simulink model "SOFIE_github_18"  (R2018a)
settings: Solver=FixedStepAuto  StartTime=0.0  StopTime=12  FixedStep=5e-6  MinStep=1e-5  RelTol=1e-3
undefined symbols (not defined in the file): start
libraries: powerlib x13, powerlib_meascontrol x5
settings Model: Creator=110198  LastModifiedBy=malinche
settings DataIOCC: ReturnWorkspaceOutputs=on
settings SFSimCC: SimUseLocalCustomCode=on
settings RTWCC: RTWUseLocalCustomCode=on

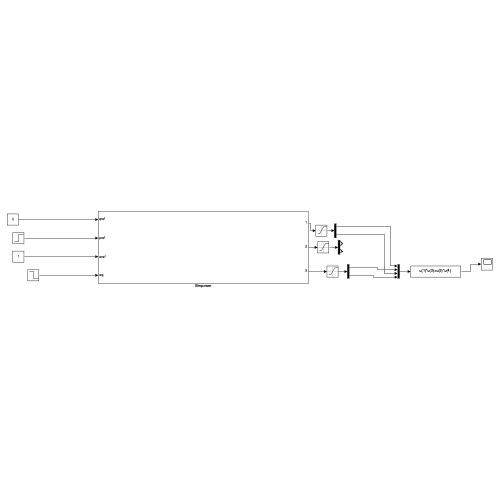
[thumbnail: Simulink's stored preview of the top-level diagram]
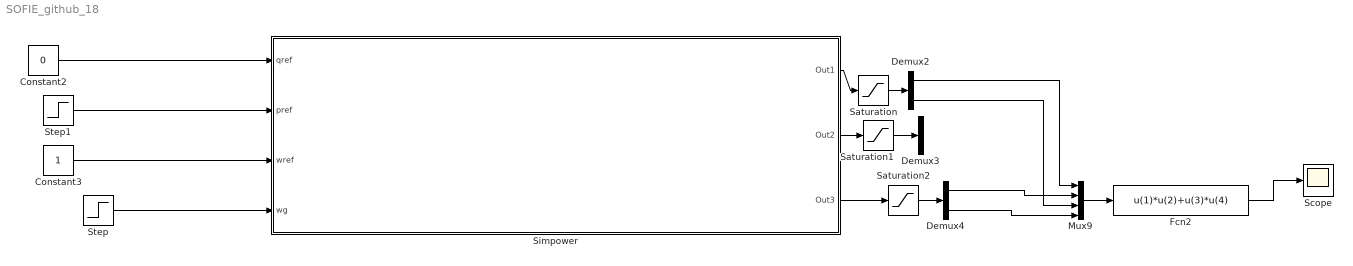
== system SOFIE_github_18 ==
  Constant2 : Constant  Value=0
  Constant3 : Constant
  Demux2 : Demux  Outputs=2
  Demux3 : Demux  Outputs=2
  Demux4 : Demux  Outputs=2
  Fcn2 : Fcn  Expr=u(1)*u(2)+u(3)*u(4)
  Mux9 : Mux
  Saturation : Saturate  UpperLimit=1.5  LowerLimit=-1.5
  Saturation1 : Saturate  UpperLimit=1.5  LowerLimit=-1.5
  Saturation2 : Saturate  UpperLimit=1.5  LowerLimit=-1.5
  Scope : Scope
  Simpower : Subsystem
  Step : Step  Time=4  Before=1  After=1-0.01  SampleTime=0
  Step1 : Step  Time=8  After=0.1  SampleTime=0
  wires:
  Step1/1 -> Simpower/2(pref)
  Constant2/1 -> Simpower/1(qref)
  Step/1 -> Simpower/4(wg)
  Constant3/1 -> Simpower/3(wref)
  Simpower/1(Out1) -> Saturation/1
  Demux2/1 -> Mux9/1
  Demux2/2 -> Mux9/3
  Simpower/2(Out2) -> Saturation1/1
  Saturation/1 -> Demux2/1
  Saturation1/1 -> Demux3/1
  Saturation2/1 -> Demux4/1
  Simpower/3(Out3) -> Saturation2/1
  Demux4/1 -> Mux9/2
  Demux4/2 -> Mux9/4
  Mux9/1 -> Fcn2/1
  Fcn2/1 -> Scope/1

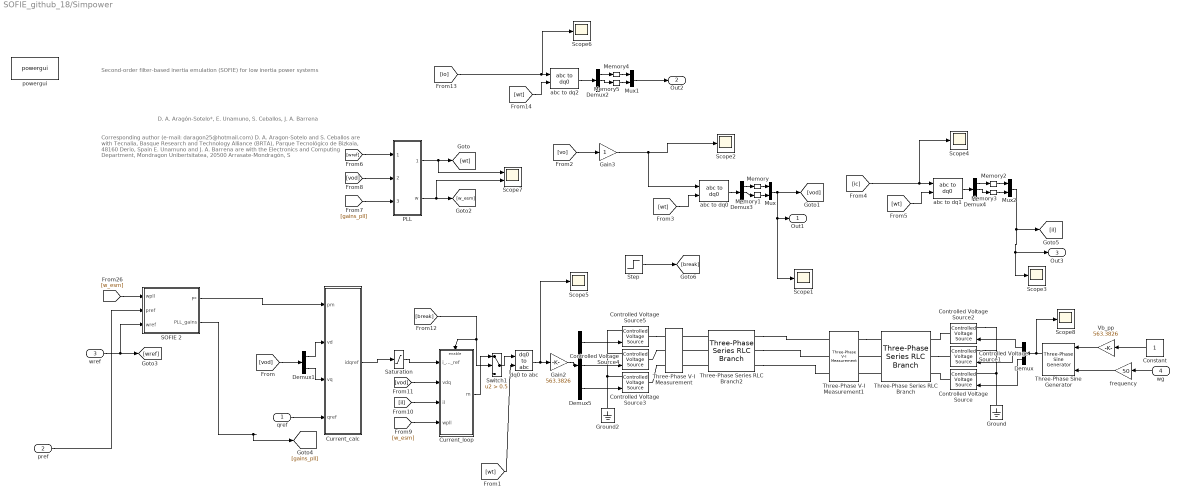
== system SOFIE_github_18/Simpower ==
  note: Second-order filter-based inertia emulation
      | (SOFIE) for low inertia power systems
  note: Corresponding author (e-mail: daragon25@hotmail.com)
      | D. A. Aragon-Sotelo and S. Ceballos are with Tecnalia, Basque Research
      | and Technology Alliance (BRTA), Parque Tecnológico de Bizkaia, 48160
      | Derio, Spain
      | E. Unamuno and J. A. Barrena are with the Electronics and Computing
      | Department, Mondragon Unibertsitatea, 20500 Arrasate-Mondragón, S
  note: D. A. Aragón-Sotelo*, E. Unamuno, S. Ceballos, J. A. Barrena
  qref : Inport
  pref : Inport  Port=2
  wref : Inport  Port=3
  wg : Inport  Port=4
  Constant : Constant
  Controlled Voltage Source{,1..5} (6 alike) : powerlib/Electrical Sources/Controlled Voltage Source  Initialize=off  Source_Type=AC  Amplitude=0  Phase=0  Frequency=0  Measurements=None
  Current_calc : Subsystem
  Current_loop : Subsystem
  Demux{,2..5} (5 alike) : Demux  Outputs=3
  Demux1 : Demux  Outputs=2
  Gain2 : Gain  Gain=563.3826
  Gain3 : Gain
  Ground : powerlib/Elements/Ground  LConnTagsString=a
  Ground2 : powerlib/Elements/Ground  LConnTagsString=a
  Memory : Memory  InitialCondition=1
  Memory1 : Memory
  Memory2 : Memory  InitialCondition=1
  Memory3 : Memory
  Memory4 : Memory  InitialCondition=1
  Memory5 : Memory
  Mux : Mux  Inputs=2
  Mux1 : Mux  Inputs=2
  Mux2 : Mux  Inputs=2
  PLL : Subsystem
  SOFIE 2 : Subsystem
  Saturation : Saturate  UpperLimit=2  LowerLimit=-2
  Scope{1..6,8} (7 alike) : Scope
  Scope7 : Scope  NumInputPorts=2
  Step : Step  Time=2  SampleTime=0
  Switch1 : Switch  Criteria=u2 > Threshold  Threshold=0.5
  Three-Phase Series RLC Branch : powerlib/Elements/Three-Phase Series RLC Branch  LConnTagsString=A|B|C  RConnTagsString=A|B|C  BranchType=RL  Resistance=0.0017  Inductance=1.6532e-05  Capacitance=1e-6  Measurements=None
  Three-Phase Series RLC Branch2 : powerlib/Elements/Three-Phase Series RLC Branch  LConnTagsString=A|B|C  RConnTagsString=A|B|C  BranchType=RL  Resistance=0.0010  Inductance=4.4086e-05  Capacitance=1e-6  Measurements=None
  Three-Phase Sine Generator : powerlib_meascontrol/Pulse & Signal Generators/Three-Phase Sine Generator  Ts=0
      settings: SourceProductBaseCode=PS
  Three-Phase V-I Measurement : powerlib/Measurements/Three-Phase V-I Measurement  VoltageMeasurement=phase-to-ground  SetLabelV=on  LabelV=Vcabc  Vpu=on  VpuLL=off  CurrentMeasurement=yes  SetLabelI=on  LabelI=ic  Ipu=on  Pbase=2.75e6  Vbase=690  OutputType=Complex  PhasorSimulation=off  PSBequivalent=0
  Three-Phase V-I Measurement1 : powerlib/Measurements/Three-Phase V-I Measurement  VoltageMeasurement=phase-to-ground  SetLabelV=on  LabelV=vo  Vpu=on  VpuLL=off  CurrentMeasurement=yes  SetLabelI=on  LabelI=io  Ipu=on  Pbase=2.75e6  Vbase=600  OutputType=Complex  PhasorSimulation=off  PSBequivalent=0
  Vb_pp : Gain  Gain=563.3826
  abc to dq0 : powerlib_meascontrol/Transformations/abc to dq0  Alignment=90 degrees behind phase A axis
  abc to dq1 : powerlib_meascontrol/Transformations/abc to dq0  Alignment=90 degrees behind phase A axis
  abc to dq2 : powerlib_meascontrol/Transformations/abc to dq0  Alignment=90 degrees behind phase A axis
  dq0 to abc : powerlib_meascontrol/Transformations/dq0 to abc  Alignment=90 degrees behind phase A axis
  frequency : Gain  Gain=50
  powergui : powerlib/powergui  Priority=1  SimulationMode=Discrete  SampleTime=20e-5  frequency=60  Iterations=50  frequencyindice=0  Pbase=100e6  ErrMax=1e-4  UnitsV=kV  UnitsW=MW  buscounter=0  FunctionMessages=off  echomessages=off  EnableUseOfTLC=off  CurrentSourceSwitches=off  DisableSnubberDevices=off  DisableRonSwitches=off  DisableVfSwitches=off  DisplayEquations=off  AutomaticDiscreteSolvers=off  SolverType=Tustin/Backward Euler (TBE)  Interpol=off  ExternalGateDelay=off  methode=off  Ts=100  x0status=blocks  SPID=on  SwTol=0  HookPort=off  NonlinearTolerance=0  nMaxIteration=15  ContinueOnMaxIteration=off  RestoreLinks=warning  ResistiveCurrentMeasurement=off  Frange=[0:2:500]  Ylog=off  Xlog=on  ShowGrid=off  save=off  variable=ZData  structure=0  ZoomFFT=off  StartTime=0.0  cycles=1  DisplayStyle=1  fundamental=60  FreqAxis=off  MaxFrequency=1000  frequencyindicesteady=1  RmsSteady=1  display=off
  Out1 : Outport  VectorParamsAs1DForOutWhenUnconnected=off
  Out2 : Outport  Port=2  VectorParamsAs1DForOutWhenUnconnected=off
  Out3 : Outport  Port=3  VectorParamsAs1DForOutWhenUnconnected=off
  wires:
  Three-Phase Sine Generator/1 -> Scope8/1, Demux/1
  Demux/1 -> Controlled Voltage Source2/1
  Demux/2 -> Controlled Voltage Source1/1
  Demux/3 -> Controlled Voltage Source/1
  Vb_pp/1 -> Three-Phase Sine Generator/1
  Constant/1 -> Vb_pp/1
  [w_esm] -> SOFIE 2/1(wpll)
  qref/1 -> Current_calc/4(qref)
  pref/1 -> SOFIE 2/2(pref)
  [vod] -> Demux1/1
  wref/1 -> SOFIE 2/3(wref), [wref]
  [wt] -> dq0 to abc/2
  [wt] -> abc to dq0/2
  frequency/1 -> Three-Phase Sine Generator/3
  wg/1 -> frequency/1
  abc to dq0/1 -> Demux3/1
  Mux/1 -> Scope1/1, Out1/1, [vod]
  Demux4/1 -> Memory2/1
  [wt] -> abc to dq1/2
  abc to dq1/1 -> Demux4/1
  Mux2/1 -> Out3/1, Scope3/1, [il]
  [wref] -> PLL/1(wref)
  SOFIE 2/2(PLL_gains) -> [gains_pll]
  [gains_pll] -> PLL/3(gains)
  [vod] -> PLL/2(vodq)
  PLL/2(w) -> Scope7/2, [w_esm]
  [w_esm] -> Current_loop/4(wpll)
  [il] -> Current_loop/3(il)
  [vod] -> Current_loop/2(vdq)
  Demux1/1 -> Current_calc/2(vd)
  Demux1/2 -> Current_calc/3(vq)
  Demux3/1 -> Memory/1
  Memory/1 -> Mux/1
  Demux3/2 -> Memory1/1
  Memory1/1 -> Mux/2
  Memory2/1 -> Mux2/1
  Demux4/2 -> Memory3/1
  Memory3/1 -> Mux2/2
  Step/1 -> [break]
  Memory4/1 -> Mux1/1
  Demux2/2 -> Memory5/1
  Demux2/1 -> Memory4/1
  abc to dq2/1 -> Demux2/1
  [wt] -> abc to dq2/2
  Mux1/1 -> Out2/1
  Memory5/1 -> Mux1/2
  Saturation/1 -> Current_loop/1(i_dq_ref)
  Current_loop/1(m) -> Switch1/1
  Switch1/1 -> dq0 to abc/1
  [break] -> Current_loop/Enable, Switch1/2
  [io] -> Scope6/1, abc to dq2/1
  [ic] -> Scope4/1, abc to dq1/1
  dq0 to abc/1 -> Scope5/1, Gain2/1
  Gain2/1 -> Demux5/1
  Gain3/1 -> abc to dq0/1, Scope2/1
  [vo] -> Gain3/1
  Demux5/1 -> Controlled Voltage Source5/1
  Demux5/2 -> Controlled Voltage Source4/1
  Demux5/3 -> Controlled Voltage Source3/1
  PLL/1(theta) -> Scope7/1, [wt]
  SOFIE 2/1(P*) -> Current_calc/1(pm)
  Current_calc/1(idqref) -> Saturation/1
  connections:
  Three-Phase Series RLC Branch/RConn2 -- Controlled Voltage Source1/RConn1
  Controlled Voltage Source/RConn1 -- Three-Phase Series RLC Branch/RConn3
  Controlled Voltage Source2/RConn1 -- Three-Phase Series RLC Branch/RConn1
  Ground/LConn1 -- Controlled Voltage Source/LConn1 -- Controlled Voltage Source2/LConn1 -- Controlled Voltage Source1/LConn1
  Three-Phase Series RLC Branch2/RConn3 -- Three-Phase V-I Measurement1/LConn3
  Three-Phase Series RLC Branch2/RConn2 -- Three-Phase V-I Measurement1/LConn2
  Three-Phase Series RLC Branch2/RConn1 -- Three-Phase V-I Measurement1/LConn1
  Three-Phase V-I Measurement1/RConn1 -- Three-Phase Series RLC Branch/LConn1
  Three-Phase Series RLC Branch/LConn2 -- Three-Phase V-I Measurement1/RConn2
  Three-Phase Series RLC Branch/LConn3 -- Three-Phase V-I Measurement1/RConn3
  Controlled Voltage Source5/RConn1 -- Three-Phase V-I Measurement/LConn1
  Three-Phase V-I Measurement/LConn2 -- Controlled Voltage Source4/RConn1
  Three-Phase V-I Measurement/LConn3 -- Controlled Voltage Source3/RConn1
  Ground2/LConn1 -- Controlled Voltage Source5/LConn1 -- Controlled Voltage Source4/LConn1 -- Controlled Voltage Source3/LConn1
  Three-Phase Series RLC Branch2/LConn1 -- Three-Phase V-I Measurement/RConn1
  Three-Phase Series RLC Branch2/LConn2 -- Three-Phase V-I Measurement/RConn2
  Three-Phase Series RLC Branch2/LConn3 -- Three-Phase V-I Measurement/RConn3

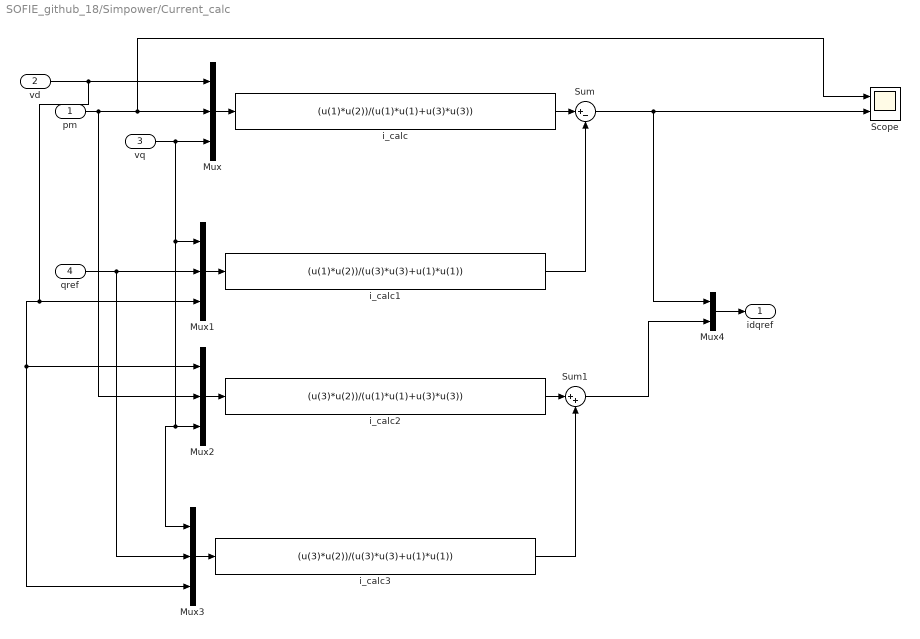
== system SOFIE_github_18/Simpower/Current_calc ==
  pm : Inport
  vd : Inport  Port=2
  vq : Inport  Port=3
  qref : Inport  Port=4
  Mux{,1..3} (4 alike) : Mux  Inputs=3
  Mux4 : Mux  Inputs=2
  Scope : Scope  NumInputPorts=2
  Sum : Sum  Inputs=|+-
  Sum1 : Sum  Inputs=|++
  i_calc : Fcn  Expr=(u(1)*u(2))/(u(1)*u(1)+u(3)*u(3))
  i_calc1 : Fcn  Expr=(u(1)*u(2))/(u(3)*u(3)+u(1)*u(1))
  i_calc2 : Fcn  Expr=(u(3)*u(2))/(u(1)*u(1)+u(3)*u(3))
  i_calc3 : Fcn  Expr=(u(3)*u(2))/(u(3)*u(3)+u(1)*u(1))
  idqref : Outport  VectorParamsAs1DForOutWhenUnconnected=off
  wires:
  Mux/1 -> i_calc/1
  i_calc/1 -> Sum/1
  i_calc1/1 -> Sum/2
  Mux1/1 -> i_calc1/1
  Sum/1 -> Mux4/1, Scope/2
  vq/1 -> Mux3/1, Mux2/3, Mux1/1, Mux/3
  Sum1/1 -> Mux4/2
  vd/1 -> Mux/1, Mux1/3, Mux2/1, Mux3/3
  i_calc2/1 -> Sum1/1
  qref/1 -> Mux1/2, Mux3/2
  Mux2/1 -> i_calc2/1
  pm/1 -> Scope/1, Mux/2, Mux2/2
  i_calc3/1 -> Sum1/2
  Mux3/1 -> i_calc3/1
  Mux4/1 -> idqref/1

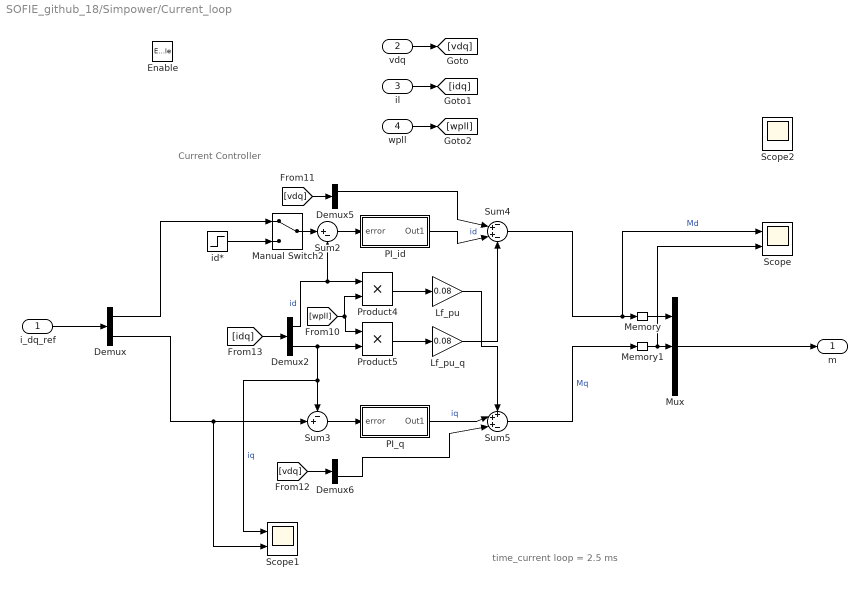
== system SOFIE_github_18/Simpower/Current_loop ==
  note: time_current loop = 2.5 ms
  note: Current Controller
  i_dq_ref : Inport
  vdq : Inport  Port=2
  il : Inport  Port=3
  wpll : Inport  Port=4
  Enable : EnablePort
  Demux{,2,5..6} (4 alike) : Demux  Outputs=2
  Lf_pu : Gain  Gain=0.08
  Lf_pu_q : Gain  Gain=0.08
  Manual Switch2 : ManualSwitch
  Memory : Memory  InitialCondition=1
  Memory1 : Memory
  Mux : Mux  Inputs=3
  PI_id : Subsystem
  PI_q : Subsystem
  Product4 : Product
  Product5 : Product
  Scope : Scope  NumInputPorts=2
  Scope1 : Scope  NumInputPorts=2
  Scope2 : Scope  NumInputPorts=2
  Sum2 : Sum  Inputs=|+-
  Sum3 : Sum  Inputs=-+|
  Sum4 : Sum  Inputs=-++-
  Sum5 : Sum  Inputs=+++-
  id* : Step  After=0  SampleTime=0
  m : Outport  VectorParamsAs1DForOutWhenUnconnected=off
  wires:
  id*/1 -> Manual Switch2/2
  [vdq] -> Demux5/1
  PI_q/1(Out1) -> Sum5/2  "iq"
  Demux2/1 -> Sum2/2, Product4/1  "id"
  [idq] -> Demux2/1
  [vdq] -> Demux6/1
  [wpll] -> Product5/1, Product4/2
  Manual Switch2/1 -> Sum2/1
  Product5/1 -> Lf_pu_q/1
  Sum2/1 -> PI_id/1(error)
  Demux/1 -> Manual Switch2/1
  Product4/1 -> Lf_pu/1
  Demux2/2 -> Scope1/1, Sum3/1, Product5/2  "iq"
  vdq/1 -> [vdq]
  il/1 -> [idq]
  wpll/1 -> [wpll]
  i_dq_ref/1 -> Demux/1
  Memory1/1 -> Scope/2, Mux/2
  Memory/1 -> Mux/1
  Mux/1 -> m/1
  Sum3/1 -> PI_q/1(error)
  Sum4/1 -> Scope/1, Memory/1  "Md"
  Sum5/1 -> Memory1/1  "Mq"
  Demux/2 -> Scope1/2, Sum3/2
  Lf_pu/1 -> Sum5/1
  Lf_pu_q/1 -> Sum4/4
  PI_id/1(Out1) -> Sum4/3  "id"
  Demux5/1 -> Sum4/2
  Demux6/2 -> Sum5/3

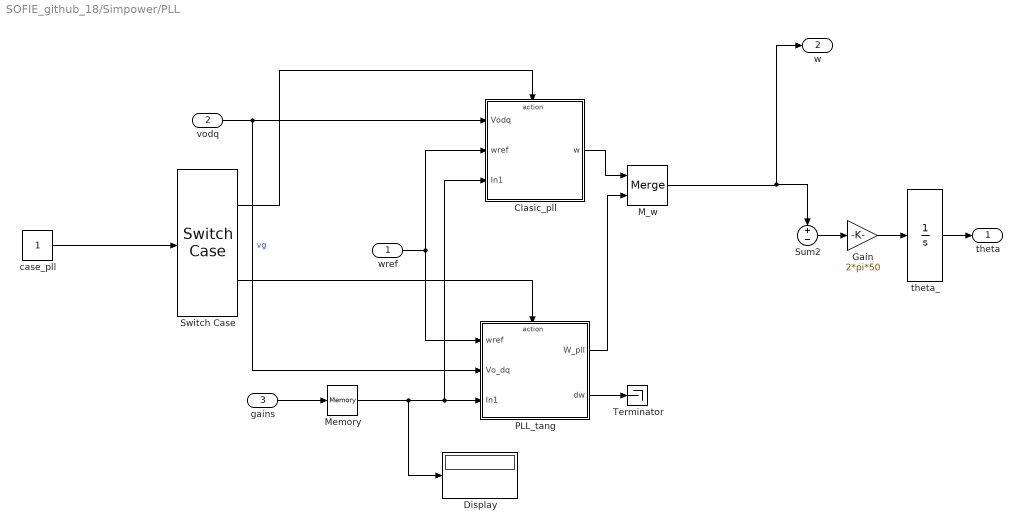
== system SOFIE_github_18/Simpower/PLL ==
  wref : Inport
  vodq : Inport  Port=2
  gains : Inport  Port=3
  Clasic_pll : Subsystem  TreatAsAtomicUnit=on
  Display : Display
  Gain : Gain  Gain=2*pi*50
  M_w : Merge
  Memory : Memory  InitialCondition=[ 0.001 0.0001]
  PLL_tang : Subsystem
  Sum2 : Sum  Inputs=+-
  Switch Case : SwitchCase  CaseConditions={1,0}  ShowDefaultCase=off
  Terminator : Terminator
  case_pll : Constant
  theta_ : Integrator  InitialCondition=-pi/2
  theta : Outport  VectorParamsAs1DForOutWhenUnconnected=off
  w : Outport  Port=2  VectorParamsAs1DForOutWhenUnconnected=off
  wires:
  PLL_tang/1(W_pll) -> M_w/2
  case_pll/1 -> Switch Case/1
  Switch Case/2 -> PLL_tang/Action
  Switch Case/1 -> Clasic_pll/Action
  wref/1 -> PLL_tang/1(wref), Clasic_pll/2(wref)
  vodq/1 -> PLL_tang/2(Vo_dq), Clasic_pll/1(Vodq)  "vg"
  Clasic_pll/1(w) -> M_w/1
  theta_/1 -> theta/1
  PLL_tang/2(dw) -> Terminator/1
  gains/1 -> Memory/1
  Memory/1 -> Display/1, PLL_tang/3(In1), Clasic_pll/3(In1)
  Sum2/1 -> Gain/1
  Gain/1 -> theta_/1
  M_w/1 -> w/1, Sum2/1

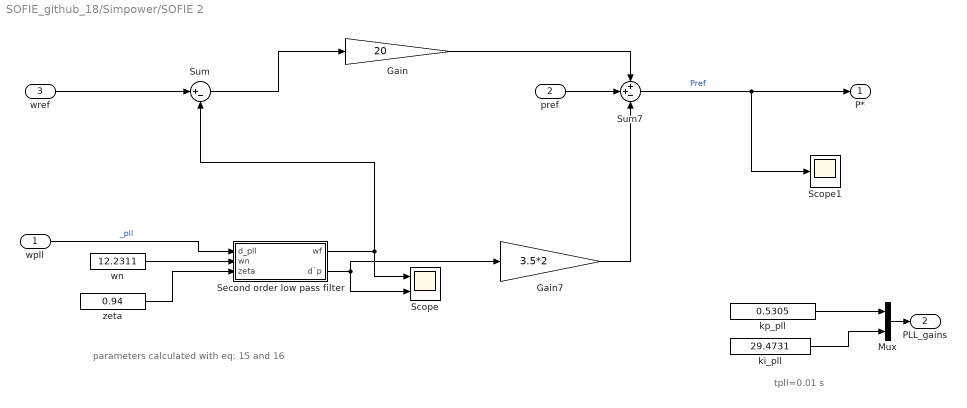
== system SOFIE_github_18/Simpower/SOFIE 2 ==
  note: parameters calculated with eq: 15 and 16
  note: tpll=0.01 s
  wpll : Inport
  pref : Inport  Port=2
  wref : Inport  Port=3
  Gain : Gain  Gain=20
  Gain7 : Gain  Gain=3.5*2
  Mux : Mux  Inputs=2
  Scope : Scope  NumInputPorts=2
  Scope1 : Scope
  Second order low pass filter : Subsystem
  Sum : Sum  Inputs=|+-
  Sum7 : Sum  Inputs=++-
  ki_pll : Constant  Value=29.4731
  kp_pll : Constant  Value=0.5305
  wn : Constant  Value=12.2311
  zeta : Constant  Value=0.94
  P* : Outport  VectorParamsAs1DForOutWhenUnconnected=off
  PLL_gains : Outport  Port=2  VectorParamsAs1DForOutWhenUnconnected=off
  wires:
  Sum7/1 -> Scope1/1, P*/1  "Pref"
  Gain/1 -> Sum7/1
  wpll/1 -> Second order low pass filter/1(d_pll)  "_pll"
  Sum/1 -> Gain/1
  wref/1 -> Sum/1
  kp_pll/1 -> Mux/1
  Mux/1 -> PLL_gains/1
  ki_pll/1 -> Mux/2
  Second order low pass filter/1(wf) -> Sum/2, Scope/1
  Second order low pass filter/2(d`p) -> Gain7/1, Scope/2
  Gain7/1 -> Sum7/3
  pref/1 -> Sum7/2
  wn/1 -> Second order low pass filter/2(wn)
  zeta/1 -> Second order low pass filter/3(zeta)

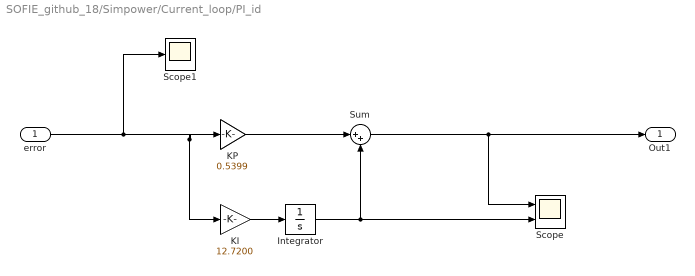
== system SOFIE_github_18/Simpower/Current_loop/PI_id ==
  error : Inport
  Integrator : Integrator  UpperSaturationLimit=1  LowerSaturationLimit=-1
  KI : Gain  Gain=12.7200
  KP : Gain  Gain=0.5399
  Scope : Scope  NumInputPorts=2
  Scope1 : Scope
  Sum : Sum  Inputs=|++
  Out1 : Outport  VectorParamsAs1DForOutWhenUnconnected=off
  wires:
  KP/1 -> Sum/1
  KI/1 -> Integrator/1
  error/1 -> Scope1/1, KI/1, KP/1
  Integrator/1 -> Sum/2, Scope/2
  Sum/1 -> Out1/1, Scope/1

== system SOFIE_github_18/Simpower/Current_loop/PI_q ==
  error : Inport
  Integrator : Integrator  UpperSaturationLimit=1  LowerSaturationLimit=-1
  KI : Gain  Gain=12.7200
  KP : Gain  Gain=0.5399
  Scope : Scope  NumInputPorts=2
  Sum : Sum  Inputs=|++
  Out1 : Outport  VectorParamsAs1DForOutWhenUnconnected=off
  wires:
  KP/1 -> Sum/1
  KI/1 -> Integrator/1
  Integrator/1 -> Scope/1, Sum/2
  error/1 -> Scope/2, KI/1, KP/1
  Sum/1 -> Out1/1

== system SOFIE_github_18/Simpower/PLL/Clasic_pll ==
  Vodq : Inport
  wref : Inport  Port=2
  In1 : Inport  Port=3
  Action Port : ActionPort
  PLL : Subsystem
  w : Outport  VectorParamsAs1DForOutWhenUnconnected=off
  wires:
  PLL/1(ws) -> w/1
  Vodq/1 -> PLL/1(Vdq+)
  wref/1 -> PLL/2(wref)
  In1/1 -> PLL/3(In1)

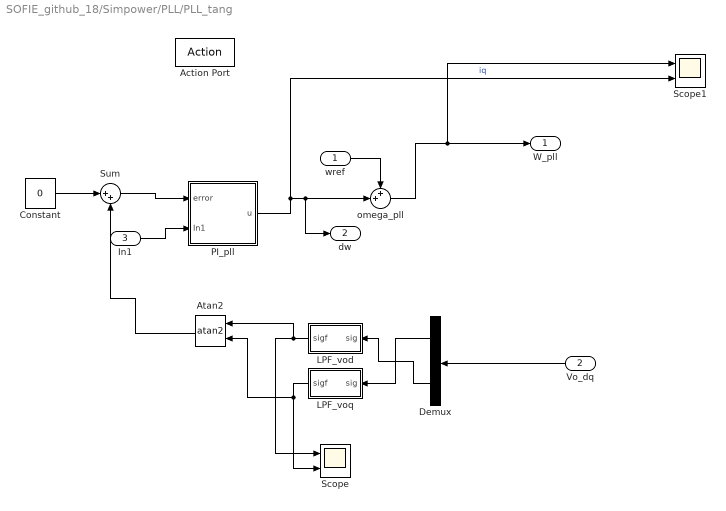
== system SOFIE_github_18/Simpower/PLL/PLL_tang ==
  wref : Inport
  Vo_dq : Inport  Port=2
  In1 : Inport  Port=3
  Action Port : ActionPort
  Atan2 : Trigonometry  Operator=atan2
  Constant : Constant  Value=0  OutDataTypeStr=double
  Demux : Demux  Outputs=2
  LPF_vod : Subsystem
  LPF_voq : Subsystem
  PI_pll : Subsystem
  Scope : Scope  NumInputPorts=2
  Scope1 : Scope  NumInputPorts=2
  Sum : Sum  Inputs=|++
  omega_pll : Sum  Inputs=++|
  W_pll : Outport  VectorParamsAs1DForOutWhenUnconnected=off
  dw : Outport  Port=2  VectorParamsAs1DForOutWhenUnconnected=off
  wires:
  Atan2/1 -> Sum/2
  Sum/1 -> PI_pll/1(error)
  PI_pll/1(u) -> Scope1/2, dw/1, omega_pll/2  "iq"
  LPF_vod/1(sigf) -> Atan2/1, Scope/1
  LPF_voq/1(sigf) -> Atan2/2, Scope/2
  Vo_dq/1 -> Demux/1
  Constant/1 -> Sum/1
  Demux/1 -> LPF_voq/1(sig)
  Demux/2 -> LPF_vod/1(sig)
  wref/1 -> omega_pll/1
  omega_pll/1 -> Scope1/1, W_pll/1
  In1/1 -> PI_pll/2(In1)

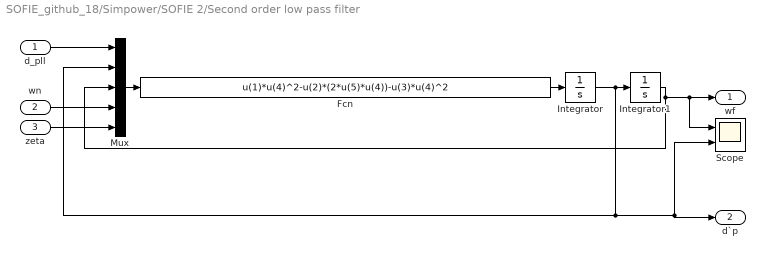
== system SOFIE_github_18/Simpower/SOFIE 2/Second order low pass filter ==
  d_pll : Inport
  wn : Inport  Port=2
  zeta : Inport  Port=3
  Fcn : Fcn  Expr=u(1)*u(4)^2-u(2)*(2*u(5)*u(4))-u(3)*u(4)^2
  Integrator : Integrator
  Integrator1 : Integrator  InitialCondition=1
  Mux : Mux  Inputs=5
  Scope : Scope  NumInputPorts=2
  wf : Outport  VectorParamsAs1DForOutWhenUnconnected=off
  d`p : Outport  Port=2  VectorParamsAs1DForOutWhenUnconnected=off
  wires:
  d_pll/1 -> Mux/1
  Mux/1 -> Fcn/1
  Fcn/1 -> Integrator/1
  Integrator/1 -> Mux/2, Scope/2, d`p/1, Integrator1/1
  Integrator1/1 -> Scope/1, wf/1, Mux/3
  wn/1 -> Mux/4
  zeta/1 -> Mux/5

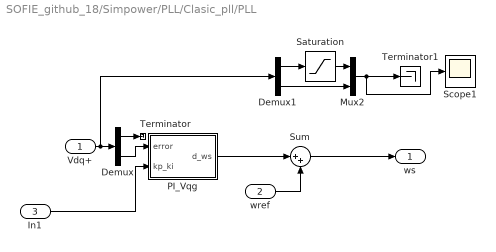
== system SOFIE_github_18/Simpower/PLL/Clasic_pll/PLL ==
  Vdq+ : Inport
  wref : Inport  Port=2
  In1 : Inport  Port=3
  Demux : Demux  Outputs=2
  Demux1 : Demux  Outputs=2
  Mux2 : Mux  Inputs=2
  PI_Vqg : Subsystem
  Saturation : Saturate  UpperLimit=inf  LowerLimit=eps
  Scope1 : Scope
  Sum : Sum  Inputs=|++
  Terminator : Terminator
  Terminator1 : Terminator
  ws : Outport  VectorParamsAs1DForOutWhenUnconnected=off
  wires:
  Demux/2 -> PI_Vqg/1(error)
  Mux2/1 -> Scope1/1, Terminator1/1
  Vdq+/1 -> Demux1/1, Demux/1
  Demux1/1 -> Saturation/1
  Saturation/1 -> Mux2/1
  Demux1/2 -> Mux2/2
  Demux/1 -> Terminator/1
  PI_Vqg/1(d_ws) -> Sum/1
  Sum/1 -> ws/1
  wref/1 -> Sum/2
  In1/1 -> PI_Vqg/2(kp_ki)

== system SOFIE_github_18/Simpower/PLL/PLL_tang/LPF_vod ==
  sig : Inport
  Fcn : Fcn  Expr=- 500*u(1) + 500*u(2)
  Integrator : Integrator
  Mux : Mux  Inputs=2
  sigf : Outport  VectorParamsAs1DForOutWhenUnconnected=off
  wires:
  Integrator/1 -> sigf/1, Mux/1
  Fcn/1 -> Integrator/1
  sig/1 -> Mux/2
  Mux/1 -> Fcn/1

== system SOFIE_github_18/Simpower/PLL/PLL_tang/LPF_voq ==
  sig : Inport
  Fcn : Fcn  Expr=- 500*u(1) +500*u(2)
  Integrator : Integrator
  Mux : Mux  Inputs=2
  sigf : Outport  VectorParamsAs1DForOutWhenUnconnected=off
  wires:
  Integrator/1 -> Mux/1, sigf/1
  Fcn/1 -> Integrator/1
  sig/1 -> Mux/2
  Mux/1 -> Fcn/1

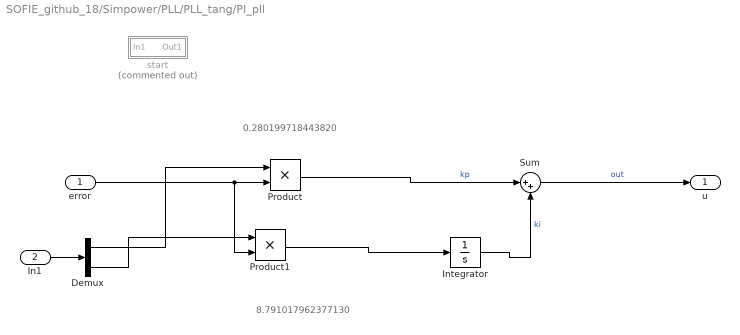
== system SOFIE_github_18/Simpower/PLL/PLL_tang/PI_pll ==
  note: 8.791017962377130
  note: 0.280199718443820
  error : Inport
  In1 : Inport  Port=2
  Demux : Demux  Outputs=2
  Integrator : Integrator
  Product : Product
  Product1 : Product
  Sum : Sum  Inputs=|++
  start : Subsystem  Commented=on
  u : Outport  VectorParamsAs1DForOutWhenUnconnected=off
  wires:
  Product/1 -> Sum/1  "kp"
  Product1/1 -> Integrator/1
  Sum/1 -> u/1  "out"
  error/1 -> Product1/2, Product/2
  Integrator/1 -> Sum/2  "ki"
  Demux/1 -> Product/1
  Demux/2 -> Product1/1
  In1/1 -> Demux/1

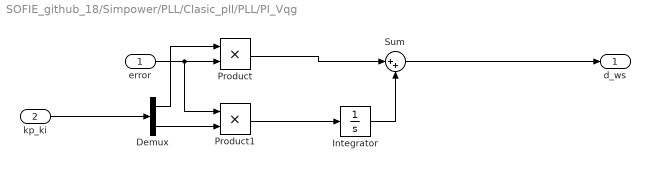
== system SOFIE_github_18/Simpower/PLL/Clasic_pll/PLL/PI_Vqg ==
  error : Inport
  kp_ki : Inport  Port=2
  Demux : Demux  Outputs=2
  Integrator : Integrator
  Product : Product
  Product1 : Product
  Sum : Sum  Inputs=|++
  d_ws : Outport  VectorParamsAs1DForOutWhenUnconnected=off
  wires:
  Product1/1 -> Integrator/1
  error/1 -> Product1/1, Product/2
  Product/1 -> Sum/1
  Sum/1 -> d_ws/1
  Integrator/1 -> Sum/2
  Demux/1 -> Product/1
  kp_ki/1 -> Demux/1
  Demux/2 -> Product1/2

== system SOFIE_github_18/Simpower/PLL/PLL_tang/PI_pll/start ==
  In1 : Inport
  Product : Product
  Step : Step  Time=start  SampleTime=0
  Out1 : Outport  VectorParamsAs1DForOutWhenUnconnected=off
  wires:
  Product/1 -> Out1/1
  In1/1 -> Product/1
  Step/1 -> Product/2
